simulink model "simu_4qc_transform2018a"  (R2018a)
settings: Solver=FixedStepAuto  StartTime=0.0  StopTime=40  FixedStep=0.01  RelTol=1e-3
InitFcn:
  | init_conditions
values from neighbouring files (symbols this model uses):
  dgaina = 4e-5    (= 4e-05)    [init_conditions.m]
  dgainb = dgaina    (= 4e-05)    [init_conditions.m]
  fd0 = [0;0;m*g/4;0;0;m*g/4;0;0;m*g/4;0;0;m*g/4]    [init_conditions.m]
  g = 9.81    [init_conditions.m]
  IB = diag([IBxy, IBxy, IBz])    [init_conditions.m]
  igaina = 0e-5    (= 0)    [init_conditions.m]
  igainb = igaina    (= 0)    [init_conditions.m]
  Lh = 0.001    [init_conditions.m]
  Lw = 0.18    [init_conditions.m]
  m = (m_qc+0.006)*4 + m_main    (= 0.156)    [init_conditions.m]
  m_main = 0.012    [init_conditions.m]
  m_qc = 0.03    [init_conditions.m]
  np = [np1; np2; np3; np4; np5; ones(numpad,1)*np5(end,:)]    [init_conditions.m]
  pgaina = 1.5e-4    (= 0.00015)    [init_conditions.m]
  pgainb = pgaina    (= 0.00015)    [init_conditions.m]
  phi = zeros(num1+num2+num3+num4+num5+numpad, 1)    [init_conditions.m]
  psi = zeros(num1+num2+num3+num4+num5+numpad, 1)    [init_conditions.m]
  StepSize = 0.01    [init_conditions.m]
  the = [zeros(1,num1+num2), th, th(end) * ones(1, num4+num5+numpad)].'    [init_conditions.m]
undefined symbols (not defined in the file or in its folder): X, Y, Z
libraries: sm_lib x51, nesl_utility x26, simulink_extras x12, simulink x8, sharedtransform x1
(part 2 of 2)

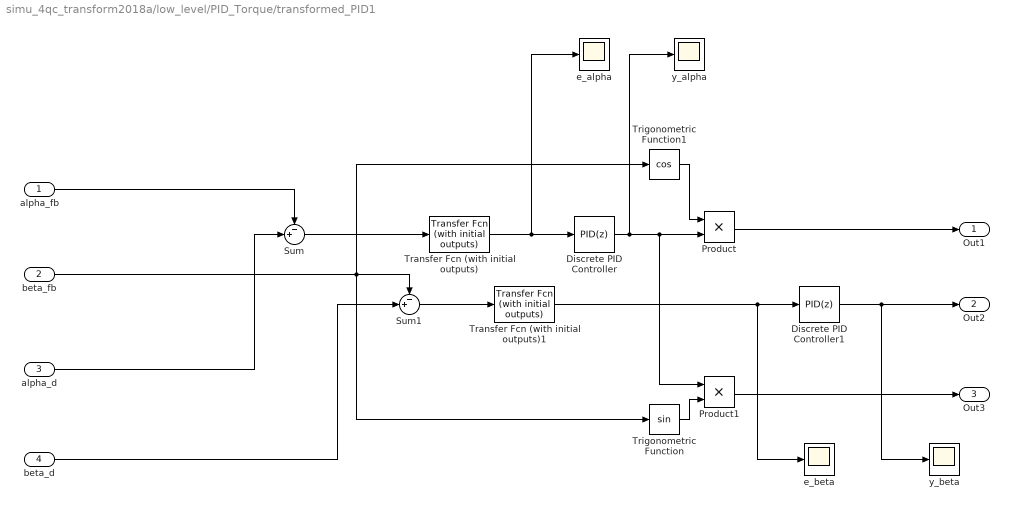
== system simu_4qc_transform2018a/low_level/PID_Torque/transformed_PID1 ==
  alpha_fb : Inport
  beta_fb : Inport  Port=2
  alpha_d : Inport  Port=3
  beta_d : Inport  Port=4
  Discrete PID Controller : simulink/Continuous/PID Controller  Controller=PID  TimeDomain=Discrete-time  SampleTime=-1  IntegratorMethod=Forward Euler  FilterMethod=Forward Euler  Form=Parallel  UseFilter=off  ControllerParametersSource=internal  P=pgaina  I=igaina  D=dgaina  N=50  InitialConditionSource=internal  InitialConditionForIntegrator=0  InitialConditionForFilter=0  ExternalReset=none  LimitOutput=off  UpperSaturationLimit=inf  LowerSaturationLimit=-inf  LinearizeAsGain=off  AntiWindupMode=none  Kb=1  TrackingMode=off  Kt=1  PParamMin=[]  PParamMax=[]  IParamMin=[]  IParamMax=[]  DParamMin=[]  DParamMax=[]  NParamMin=[]  NParamMax=[]  KbParamMin=[]  KbParamMax=[]  KtParamMin=[]  KtParamMax=[]  POutMin=[]  POutMax=[]  IOutMin=[]  IOutMax=[]  DOutMin=[]  DOutMax=[]  NOutMin=[]  NOutMax=[]  KbOutMin=[]  KbOutMax=[]  KtOutMin=[]  KtOutMax=[]  IntegratorOutMin=[]  IntegratorOutMax=[]  FilterOutMin=[]  FilterOutMax=[]  SumOutMin=[]  SumOutMax=[]  SumI1OutMin=[]  SumI1OutMax=[]  SumI2OutMin=[]  SumI2OutMax=[]  SumI3OutMin=[]  SumI3OutMax=[]  SumDOutMin=[]  SumDOutMax=[]  SaturationOutMin=[]  SaturationOutMax=[]  IntegratorContinuousStateAttributes=''  IntegratorStateMustResolveToSignalObject=off  IntegratorRTWStateStorageClass=Auto  FilterContinuousStateAttributes=''  FilterStateMustResolveToSignalObject=off  FilterRTWStateStorageClass=Auto  DifferentiatorICPrevScaledInput=0  DifferentiatorOutMin=[]  DifferentiatorOutMax=[]  FilterDiffOutCoefMin=[]  FilterDiffOutCoefMax=[]  SumDenOutMin=[]  SumDenOutMax=[]  SumNumOutMin=[]  SumNumOutMax=[]  ReciprocalOutMin=[]  ReciprocalOutMax=[]  DivideOutMin=[]  DivideOutMax=[]  TunerSelectOption=Transfer Function Based (PID Tuner App)
  Discrete PID Controller1 : simulink/Continuous/PID Controller  Controller=PID  TimeDomain=Discrete-time  SampleTime=-1  IntegratorMethod=Forward Euler  FilterMethod=Forward Euler  Form=Parallel  UseFilter=off  ControllerParametersSource=internal  P=pgainb  I=igainb  D=dgainb  N=50  InitialConditionSource=internal  InitialConditionForIntegrator=0  InitialConditionForFilter=0  ExternalReset=none  LimitOutput=off  UpperSaturationLimit=inf  LowerSaturationLimit=-inf  LinearizeAsGain=off  AntiWindupMode=none  Kb=1  TrackingMode=off  Kt=1  PParamMin=[]  PParamMax=[]  IParamMin=[]  IParamMax=[]  DParamMin=[]  DParamMax=[]  NParamMin=[]  NParamMax=[]  KbParamMin=[]  KbParamMax=[]  KtParamMin=[]  KtParamMax=[]  POutMin=[]  POutMax=[]  IOutMin=[]  IOutMax=[]  DOutMin=[]  DOutMax=[]  NOutMin=[]  NOutMax=[]  KbOutMin=[]  KbOutMax=[]  KtOutMin=[]  KtOutMax=[]  IntegratorOutMin=[]  IntegratorOutMax=[]  FilterOutMin=[]  FilterOutMax=[]  SumOutMin=[]  SumOutMax=[]  SumI1OutMin=[]  SumI1OutMax=[]  SumI2OutMin=[]  SumI2OutMax=[]  SumI3OutMin=[]  SumI3OutMax=[]  SumDOutMin=[]  SumDOutMax=[]  SaturationOutMin=[]  SaturationOutMax=[]  IntegratorContinuousStateAttributes=''  IntegratorStateMustResolveToSignalObject=off  IntegratorRTWStateStorageClass=Auto  FilterContinuousStateAttributes=''  FilterStateMustResolveToSignalObject=off  FilterRTWStateStorageClass=Auto  DifferentiatorICPrevScaledInput=0  DifferentiatorOutMin=[]  DifferentiatorOutMax=[]  FilterDiffOutCoefMin=[]  FilterDiffOutCoefMax=[]  SumDenOutMin=[]  SumDenOutMax=[]  SumNumOutMin=[]  SumNumOutMax=[]  ReciprocalOutMin=[]  ReciprocalOutMax=[]  DivideOutMin=[]  DivideOutMax=[]  TunerSelectOption=Transfer Function Based (PID Tuner App)
  Product : Product
  Product1 : Product
  Sum : Sum  Inputs=-+|
  Sum1 : Sum  Inputs=-+|
  Transfer Fcn (with initial outputs) : simulink_extras/Additional Linear/Transfer Fcn (with initial outputs)  N=[1]  D="[0.02  1]"  Y0=0  U0=0
  Transfer Fcn (with initial outputs)1 : simulink_extras/Additional Linear/Transfer Fcn (with initial outputs)  N=[1]  D="[0.02  1]"  Y0=0  U0=0
  Trigonometric Function : Trigonometry  OutputSignalType=real
  Trigonometric Function1 : Trigonometry  Operator=cos  OutputSignalType=real
  e_alpha : Scope
  e_beta : Scope
  y_alpha : Scope
  y_beta : Scope
  Out1 : Outport
  Out2 : Outport  Port=2
  Out3 : Outport  Port=3
  wires:
  Trigonometric Function1/1 -> Product/1
  beta_fb/1 -> Sum1/1, Trigonometric Function1/1, Trigonometric Function/1
  Discrete PID Controller1/1 -> y_beta/1, Out2/1
  Sum1/1 -> Transfer Fcn (with initial outputs)1/1
  alpha_fb/1 -> Sum/1
  alpha_d/1 -> Sum/2
  Sum/1 -> Transfer Fcn (with initial outputs)/1
  Trigonometric Function/1 -> Product1/2
  beta_d/1 -> Sum1/2
  Product1/1 -> Out3/1
  Product/1 -> Out1/1
  Discrete PID Controller/1 -> y_alpha/1, Product1/1, Product/2
  Transfer Fcn (with initial outputs)/1 -> e_alpha/1, Discrete PID Controller/1
  Transfer Fcn (with initial outputs)1/1 -> e_beta/1, Discrete PID Controller1/1

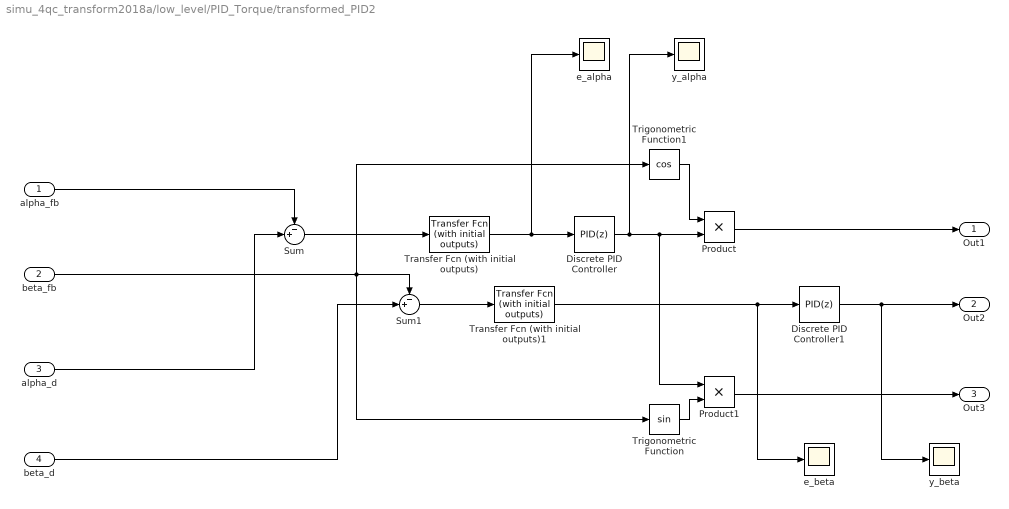
== system simu_4qc_transform2018a/low_level/PID_Torque/transformed_PID2 ==
  alpha_fb : Inport
  beta_fb : Inport  Port=2
  alpha_d : Inport  Port=3
  beta_d : Inport  Port=4
  Discrete PID Controller : simulink/Continuous/PID Controller  Controller=PID  TimeDomain=Discrete-time  SampleTime=-1  IntegratorMethod=Forward Euler  FilterMethod=Forward Euler  Form=Parallel  UseFilter=off  ControllerParametersSource=internal  P=pgaina  I=igaina  D=dgaina  N=50  InitialConditionSource=internal  InitialConditionForIntegrator=0  InitialConditionForFilter=0  ExternalReset=none  LimitOutput=off  UpperSaturationLimit=inf  LowerSaturationLimit=-inf  LinearizeAsGain=off  AntiWindupMode=none  Kb=1  TrackingMode=off  Kt=1  PParamMin=[]  PParamMax=[]  IParamMin=[]  IParamMax=[]  DParamMin=[]  DParamMax=[]  NParamMin=[]  NParamMax=[]  KbParamMin=[]  KbParamMax=[]  KtParamMin=[]  KtParamMax=[]  POutMin=[]  POutMax=[]  IOutMin=[]  IOutMax=[]  DOutMin=[]  DOutMax=[]  NOutMin=[]  NOutMax=[]  KbOutMin=[]  KbOutMax=[]  KtOutMin=[]  KtOutMax=[]  IntegratorOutMin=[]  IntegratorOutMax=[]  FilterOutMin=[]  FilterOutMax=[]  SumOutMin=[]  SumOutMax=[]  SumI1OutMin=[]  SumI1OutMax=[]  SumI2OutMin=[]  SumI2OutMax=[]  SumI3OutMin=[]  SumI3OutMax=[]  SumDOutMin=[]  SumDOutMax=[]  SaturationOutMin=[]  SaturationOutMax=[]  IntegratorContinuousStateAttributes=''  IntegratorStateMustResolveToSignalObject=off  IntegratorRTWStateStorageClass=Auto  FilterContinuousStateAttributes=''  FilterStateMustResolveToSignalObject=off  FilterRTWStateStorageClass=Auto  DifferentiatorICPrevScaledInput=0  DifferentiatorOutMin=[]  DifferentiatorOutMax=[]  FilterDiffOutCoefMin=[]  FilterDiffOutCoefMax=[]  SumDenOutMin=[]  SumDenOutMax=[]  SumNumOutMin=[]  SumNumOutMax=[]  ReciprocalOutMin=[]  ReciprocalOutMax=[]  DivideOutMin=[]  DivideOutMax=[]  TunerSelectOption=Transfer Function Based (PID Tuner App)
  Discrete PID Controller1 : simulink/Continuous/PID Controller  Controller=PID  TimeDomain=Discrete-time  SampleTime=-1  IntegratorMethod=Forward Euler  FilterMethod=Forward Euler  Form=Parallel  UseFilter=off  ControllerParametersSource=internal  P=pgainb  I=igainb  D=dgainb  N=50  InitialConditionSource=internal  InitialConditionForIntegrator=0  InitialConditionForFilter=0  ExternalReset=none  LimitOutput=off  UpperSaturationLimit=inf  LowerSaturationLimit=-inf  LinearizeAsGain=off  AntiWindupMode=none  Kb=1  TrackingMode=off  Kt=1  PParamMin=[]  PParamMax=[]  IParamMin=[]  IParamMax=[]  DParamMin=[]  DParamMax=[]  NParamMin=[]  NParamMax=[]  KbParamMin=[]  KbParamMax=[]  KtParamMin=[]  KtParamMax=[]  POutMin=[]  POutMax=[]  IOutMin=[]  IOutMax=[]  DOutMin=[]  DOutMax=[]  NOutMin=[]  NOutMax=[]  KbOutMin=[]  KbOutMax=[]  KtOutMin=[]  KtOutMax=[]  IntegratorOutMin=[]  IntegratorOutMax=[]  FilterOutMin=[]  FilterOutMax=[]  SumOutMin=[]  SumOutMax=[]  SumI1OutMin=[]  SumI1OutMax=[]  SumI2OutMin=[]  SumI2OutMax=[]  SumI3OutMin=[]  SumI3OutMax=[]  SumDOutMin=[]  SumDOutMax=[]  SaturationOutMin=[]  SaturationOutMax=[]  IntegratorContinuousStateAttributes=''  IntegratorStateMustResolveToSignalObject=off  IntegratorRTWStateStorageClass=Auto  FilterContinuousStateAttributes=''  FilterStateMustResolveToSignalObject=off  FilterRTWStateStorageClass=Auto  DifferentiatorICPrevScaledInput=0  DifferentiatorOutMin=[]  DifferentiatorOutMax=[]  FilterDiffOutCoefMin=[]  FilterDiffOutCoefMax=[]  SumDenOutMin=[]  SumDenOutMax=[]  SumNumOutMin=[]  SumNumOutMax=[]  ReciprocalOutMin=[]  ReciprocalOutMax=[]  DivideOutMin=[]  DivideOutMax=[]  TunerSelectOption=Transfer Function Based (PID Tuner App)
  Product : Product
  Product1 : Product
  Sum : Sum  Inputs=-+|
  Sum1 : Sum  Inputs=-+|
  Transfer Fcn (with initial outputs) : simulink_extras/Additional Linear/Transfer Fcn (with initial outputs)  N=[1]  D="[0.02  1]"  Y0=0  U0=0
  Transfer Fcn (with initial outputs)1 : simulink_extras/Additional Linear/Transfer Fcn (with initial outputs)  N=[1]  D="[0.02  1]"  Y0=0  U0=0
  Trigonometric Function : Trigonometry  OutputSignalType=real
  Trigonometric Function1 : Trigonometry  Operator=cos  OutputSignalType=real
  e_alpha : Scope
  e_beta : Scope
  y_alpha : Scope
  y_beta : Scope
  Out1 : Outport
  Out2 : Outport  Port=2
  Out3 : Outport  Port=3
  wires:
  Trigonometric Function1/1 -> Product/1
  beta_fb/1 -> Sum1/1, Trigonometric Function1/1, Trigonometric Function/1
  Discrete PID Controller1/1 -> y_beta/1, Out2/1
  Sum1/1 -> Transfer Fcn (with initial outputs)1/1
  alpha_fb/1 -> Sum/1
  alpha_d/1 -> Sum/2
  Sum/1 -> Transfer Fcn (with initial outputs)/1
  Trigonometric Function/1 -> Product1/2
  beta_d/1 -> Sum1/2
  Product1/1 -> Out3/1
  Product/1 -> Out1/1
  Discrete PID Controller/1 -> y_alpha/1, Product1/1, Product/2
  Transfer Fcn (with initial outputs)/1 -> e_alpha/1, Discrete PID Controller/1
  Transfer Fcn (with initial outputs)1/1 -> e_beta/1, Discrete PID Controller1/1

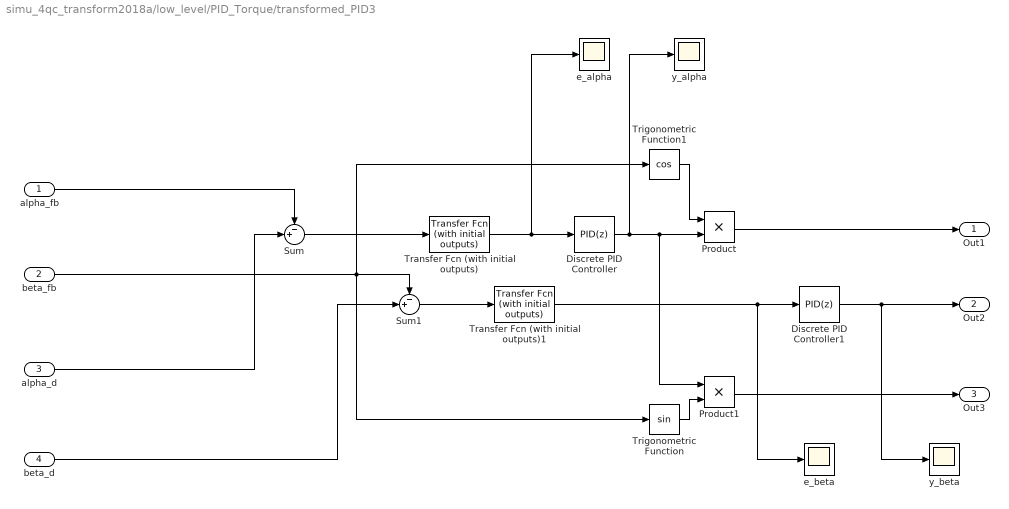
== system simu_4qc_transform2018a/low_level/PID_Torque/transformed_PID3 ==
  alpha_fb : Inport
  beta_fb : Inport  Port=2
  alpha_d : Inport  Port=3
  beta_d : Inport  Port=4
  Discrete PID Controller : simulink/Continuous/PID Controller  Controller=PID  TimeDomain=Discrete-time  SampleTime=-1  IntegratorMethod=Forward Euler  FilterMethod=Forward Euler  Form=Parallel  UseFilter=off  ControllerParametersSource=internal  P=pgaina  I=igaina  D=dgaina  N=50  InitialConditionSource=internal  InitialConditionForIntegrator=0  InitialConditionForFilter=0  ExternalReset=none  LimitOutput=off  UpperSaturationLimit=inf  LowerSaturationLimit=-inf  LinearizeAsGain=off  AntiWindupMode=none  Kb=1  TrackingMode=off  Kt=1  PParamMin=[]  PParamMax=[]  IParamMin=[]  IParamMax=[]  DParamMin=[]  DParamMax=[]  NParamMin=[]  NParamMax=[]  KbParamMin=[]  KbParamMax=[]  KtParamMin=[]  KtParamMax=[]  POutMin=[]  POutMax=[]  IOutMin=[]  IOutMax=[]  DOutMin=[]  DOutMax=[]  NOutMin=[]  NOutMax=[]  KbOutMin=[]  KbOutMax=[]  KtOutMin=[]  KtOutMax=[]  IntegratorOutMin=[]  IntegratorOutMax=[]  FilterOutMin=[]  FilterOutMax=[]  SumOutMin=[]  SumOutMax=[]  SumI1OutMin=[]  SumI1OutMax=[]  SumI2OutMin=[]  SumI2OutMax=[]  SumI3OutMin=[]  SumI3OutMax=[]  SumDOutMin=[]  SumDOutMax=[]  SaturationOutMin=[]  SaturationOutMax=[]  IntegratorContinuousStateAttributes=''  IntegratorStateMustResolveToSignalObject=off  IntegratorRTWStateStorageClass=Auto  FilterContinuousStateAttributes=''  FilterStateMustResolveToSignalObject=off  FilterRTWStateStorageClass=Auto  DifferentiatorICPrevScaledInput=0  DifferentiatorOutMin=[]  DifferentiatorOutMax=[]  FilterDiffOutCoefMin=[]  FilterDiffOutCoefMax=[]  SumDenOutMin=[]  SumDenOutMax=[]  SumNumOutMin=[]  SumNumOutMax=[]  ReciprocalOutMin=[]  ReciprocalOutMax=[]  DivideOutMin=[]  DivideOutMax=[]  TunerSelectOption=Transfer Function Based (PID Tuner App)
  Discrete PID Controller1 : simulink/Continuous/PID Controller  Controller=PID  TimeDomain=Discrete-time  SampleTime=-1  IntegratorMethod=Forward Euler  FilterMethod=Forward Euler  Form=Parallel  UseFilter=off  ControllerParametersSource=internal  P=pgainb  I=igainb  D=dgainb  N=50  InitialConditionSource=internal  InitialConditionForIntegrator=0  InitialConditionForFilter=0  ExternalReset=none  LimitOutput=off  UpperSaturationLimit=inf  LowerSaturationLimit=-inf  LinearizeAsGain=off  AntiWindupMode=none  Kb=1  TrackingMode=off  Kt=1  PParamMin=[]  PParamMax=[]  IParamMin=[]  IParamMax=[]  DParamMin=[]  DParamMax=[]  NParamMin=[]  NParamMax=[]  KbParamMin=[]  KbParamMax=[]  KtParamMin=[]  KtParamMax=[]  POutMin=[]  POutMax=[]  IOutMin=[]  IOutMax=[]  DOutMin=[]  DOutMax=[]  NOutMin=[]  NOutMax=[]  KbOutMin=[]  KbOutMax=[]  KtOutMin=[]  KtOutMax=[]  IntegratorOutMin=[]  IntegratorOutMax=[]  FilterOutMin=[]  FilterOutMax=[]  SumOutMin=[]  SumOutMax=[]  SumI1OutMin=[]  SumI1OutMax=[]  SumI2OutMin=[]  SumI2OutMax=[]  SumI3OutMin=[]  SumI3OutMax=[]  SumDOutMin=[]  SumDOutMax=[]  SaturationOutMin=[]  SaturationOutMax=[]  IntegratorContinuousStateAttributes=''  IntegratorStateMustResolveToSignalObject=off  IntegratorRTWStateStorageClass=Auto  FilterContinuousStateAttributes=''  FilterStateMustResolveToSignalObject=off  FilterRTWStateStorageClass=Auto  DifferentiatorICPrevScaledInput=0  DifferentiatorOutMin=[]  DifferentiatorOutMax=[]  FilterDiffOutCoefMin=[]  FilterDiffOutCoefMax=[]  SumDenOutMin=[]  SumDenOutMax=[]  SumNumOutMin=[]  SumNumOutMax=[]  ReciprocalOutMin=[]  ReciprocalOutMax=[]  DivideOutMin=[]  DivideOutMax=[]  TunerSelectOption=Transfer Function Based (PID Tuner App)
  Product : Product
  Product1 : Product
  Sum : Sum  Inputs=-+|
  Sum1 : Sum  Inputs=-+|
  Transfer Fcn (with initial outputs) : simulink_extras/Additional Linear/Transfer Fcn (with initial outputs)  N=[1]  D="[0.02  1]"  Y0=0  U0=0
  Transfer Fcn (with initial outputs)1 : simulink_extras/Additional Linear/Transfer Fcn (with initial outputs)  N=[1]  D="[0.02  1]"  Y0=0  U0=0
  Trigonometric Function : Trigonometry  OutputSignalType=real
  Trigonometric Function1 : Trigonometry  Operator=cos  OutputSignalType=real
  e_alpha : Scope
  e_beta : Scope
  y_alpha : Scope
  y_beta : Scope
  Out1 : Outport
  Out2 : Outport  Port=2
  Out3 : Outport  Port=3
  wires:
  Trigonometric Function1/1 -> Product/1
  beta_fb/1 -> Sum1/1, Trigonometric Function1/1, Trigonometric Function/1
  Discrete PID Controller1/1 -> y_beta/1, Out2/1
  Sum1/1 -> Transfer Fcn (with initial outputs)1/1
  alpha_fb/1 -> Sum/1
  alpha_d/1 -> Sum/2
  Sum/1 -> Transfer Fcn (with initial outputs)/1
  Trigonometric Function/1 -> Product1/2
  beta_d/1 -> Sum1/2
  Product1/1 -> Out3/1
  Product/1 -> Out1/1
  Discrete PID Controller/1 -> y_alpha/1, Product1/1, Product/2
  Transfer Fcn (with initial outputs)/1 -> e_alpha/1, Discrete PID Controller/1
  Transfer Fcn (with initial outputs)1/1 -> e_beta/1, Discrete PID Controller1/1

== matlab function simu_4qc_transform2018a/MATLAB Function ==
  data: p input; u1 output; p_dot input; R input; pr input; ep output; fr output; m parameter
function [u1, ep, fr] = position_controller(p, p_dot, R, pr, m)

kp = 3;
kv = 2;

Kp = kp * diag([1,1,3]);
Kv = kv * diag([1,1,3]);

ep = p - pr;
ev = p_dot;

% force in {I} frame
fr = m*(9.81*[0;0;1] - Kp*ep - Kv*ev);

% force in {B} frame
u1 = R.' * fr;

== matlab function simu_4qc_transform2018a/Subsystem/MATLAB Function ==
  data: Rin input; Rout output
function Rout = y_coord_180(Rin)

% % y z reversed, x same
% Rout = diag([1,-1,-1])*Rin*diag([1,-1,-1]);

% all x y z reversed
Rout = Rin.';

== matlab function simu_4qc_transform2018a/MATLAB Function1 ==
  data: R input; u2 output; O input; Rr input; eR output; Lh parameter; m parameter; IB parameter; eRiin input; eRiout output
function [u2, eR, eRiout] = attitude_controller(R, O, Rr, Lh, m, IB, eRiin)

kR = 0.5e-2;
kw = 0.5e-2;
ki = 0.3e-5;

KR = kR * diag([1,1,0.2]);
Kw = kw * diag([1,1,0.2]);
Ki = ki * diag([1,1,0.2]);

E = 1/2*(Rr.'*R - R.'*Rr);
eR = [E(3,2) E(1,3) E(2,1)]';
ew = O;
eRiout = eRiin + eR;

% Physical dynamics to cancel
rho = [0,0,-Lh].';
h = cross(O, IB * O);
tau_g = - m * 9.81 * cross(rho, R.'*[0;0;1]);

u2 = h - tau_g - KR*eR - Kw*ew - Ki*eRiin;

== matlab function simu_4qc_transform2018a/MATLAB Function2 ==
  data: u1 input; fd output; u2 input; Lw parameter; t input; StepSize parameter; the parameter
function fd = wrench_mapper(u1, u2, Lw, t, StepSize, the)

% distance from O_B to O_i
BP1 = [ Lw   0  0]';
BP2 = [  0  Lw  0]';
BP3 = [-Lw   0  0]';
BP4 = [  0 -Lw  0]';

% bijection
BP1x = [0,-BP1(3),BP1(2); BP1(3),0,-BP1(1); -BP1(2),BP1(1),0];
BP2x = [0,-BP2(3),BP2(2); BP2(3),0,-BP2(1); -BP2(2),BP2(1),0];
BP3x = [0,-BP3(3),BP3(2); BP3(3),0,-BP3(1); -BP3(2),BP3(1),0];
BP4x = [0,-BP4(3),BP4(2); BP4(3),0,-BP4(1); -BP4(2),BP4(1),0];

% compile A matrix 
A = [eye(3),eye(3),eye(3),eye(3);BP1x,BP2x,BP3x,BP4x];

% Ar maps u to q expressed in {i}
B1R = eye(3);
B2R = [ 0 -1 0;  1  0 0; 0 0 1];
B3R = [-1  0 0;  0 -1 0; 0 0 1];
B4R = [ 0  1 0; -1  0 0; 0 0 1];
Ar = A * [B1R,zeros(3,9); zeros(3,3),B2R,zeros(3,6); zeros(3,6),B3R,zeros(3,3); zeros(3,9),B4R];

td = floor(t/StepSize + 1);
marg = 0.2; %0.27;
if abs(the(td)) > (1.57-marg) && abs(the(td)) < (1.57+marg)
    Arr = [Ar(:,1),Ar(:,3:7),Ar(:,9:end)];
    ArTr = Arr.'*((Arr*Arr.')^(-1));
    
    qr = ArTr*[u1;u2];
    fd = [qr(1);0;qr(2:6);0;qr(7:end)];
    
else
    ArT = Ar.'*((Ar*Ar.')^(-1));
    fd = ArT * [u1;u2];
    
end

== matlab function simu_4qc_transform2018a/MATLAB Function5 ==
  data: F output; fd input; alpha_all output; beta_all output; fd_prev input; alpha_prev input; beta_prev input
function [F, alpha_all, beta_all] = qc_servo(fd, fd_prev, alpha_prev, beta_prev)


% ======= inverse kinematics ======
Xhat = [1 0 0]';
Yhat = [0 1 0]';

F = zeros(4,1);
alpha_all = zeros(4,1);
beta_all = zeros(4,1);

for i=1:4
    
    aprev = alpha_prev(i);
    bprev = beta_prev(i);
    
    % Desired and previous thrust direction (break 12x1 into 4 x 3x1)
    fdi = fd(3*i-2:3*i);
    fdi_prev = fd_prev(3*i-2:3*i);
    
    % force F
    F(i) = norm(fdi);
    
    tstar = fdi / norm(fdi);
    tprev = fdi_prev / norm(fdi_prev);
    
    % previous shaft axis
    sp = [0; -tprev(3); tprev(2)];
    
    % current shaft axis
    sc = [0; -tstar(3); tstar(2)];
    
    % Calc alpha inc between shaft rotations... [rad]
    ainc = atan2(norm(cross(sp,sc)), dot(sp,sc));
    
    %     ainc = 0; REDUCTION%
    
    % Determine direction (sign) of alpha_inc
    asign = sign(dot(cross(sp, sc), Xhat));
    
    % Rotate tprev about Xhat by PREVIOUS alpha_i
    Rx = [1 0 0; 0 cos(aprev) sin(aprev); 0 -sin(aprev) cos(aprev)];
    tp = Rx * tprev;
    
    % THEN update alpha_i (to current/new); Code order is important
    alpha = aprev + asign*ainc;
    
    % Rotate t_star about Xhat by CURRENT alpha_i
    Rxn = [1 0 0; 0 cos(alpha) sin(alpha); 0 -sin(alpha) cos(alpha)];
    tn = Rxn * tstar;
    
    % Find angle between "alpha-cancelled" vectors
    binc = atan2(norm(cross(tp,tn)), dot(tp,tn));
    
    % Determine direction (sign) of beta_inc
    bsign = sign(dot(cross(tp, tn), Yhat));
    
    % Update beta_i
    beta = bprev + bsign*binc;
    
    alpha_all(i) = alpha;
    beta_all(i) = beta;
    
end

== matlab function simu_4qc_transform2018a/MATLAB Function4 ==
  data: pr output; t input; np parameter; phi parameter; the parameter; psi parameter; Rr output; StepSize parameter; rotr output
function [pr, Rr, rotr] = program_trajectory(t, np, phi, the, psi, StepSize)

td = floor(t/StepSize + 1);

pr = np(td,:).';

Rx = [1 0 0; 0 cos(phi(td)) -sin(phi(td)); 0 sin(phi(td)) cos(phi(td))];
Ry = [cos(the(td)) 0 sin(the(td)); 0 1 0; -sin(the(td)) 0 cos(the(td))];
Rz = [cos(psi(td)) -sin(psi(td)) 0; sin(psi(td)) cos(psi(td)) 0; 0 0 1];
Rr = Rx * Ry * Rz;

rotr = [phi(td); the(td); psi(td)];

== matlab function simu_4qc_transform2018a/MATLAB Function3 ==
  data: f_d input; thrust output; alpha_d input; beta_d input; alpha output; beta output
function [thrust, alpha, beta] = pyAPI(f_d, alpha_d, beta_d)

thrust = 20000;
alpha = alpha_d(1);
beta = beta_d(1);
